simulink model "zerodiv01"  (Simulink 7.8)
settings: Solver=FixedStepDiscrete  StartTime=0.0  StopTime=10.0  FixedStep=Auto  RelTol=1e-3
settings Model: Creator=itoy  LastModifiedBy=itoy
settings DataIOCC: LimitDataPoints=off  SaveFormat=StructureWithTime  SaveOutput=off  SaveTime=off
settings OptimizationCC: OptimizeModelRefInitCode=on  LifeSpan=1
settings DebuggingCC: StrictBusMsg=Warning
settings RTWCC: SystemTargetFile=ert.tlc  GenCodeOnly=on  TemplateMakefile=ert_default_tmf  Description=Real-Time Workshop Embedded Coder  GenerateReport=on  ProcessScript=ert_make_rtw_hook  IncludeHyperlinkInReport=on  LaunchReport=on  GenerateTraceInfo=on  GenerateTraceReport=on  GenerateTraceReportSl=on  GenerateTraceReportSf=on  GenerateTraceReportEml=on
settings CodeAppCC: IgnoreCustomStorageClasses=off
settings ERTTargetCC: MultiwordLength=2048  GenerateSampleERTMain=on  ERTCustomFileTemplate=example_file_process.tlc  ConvertIfToSwitch=off  SuppressUnreachableDefaultCases=off

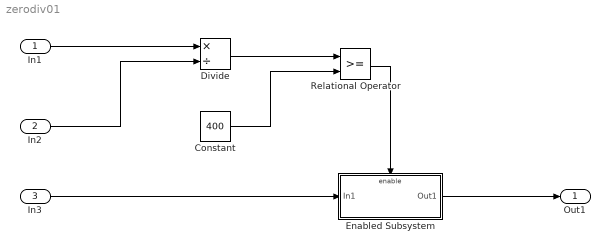
== system zerodiv01 ==
  In1 : Inport  OutMin=2  OutMax=10  OutDataTypeStr=int8
      settings: AttributesFormatString=[%<OutMax> %<OutMin>]
  In2 : Inport  Port=2  OutMin=-5  OutMax=5  OutDataTypeStr=int8
      settings: AttributesFormatString=[%<OutMax> %<OutMin>]
  In3 : Inport  Port=3  OutMin=-100  OutMax=100  OutDataTypeStr=int8
      settings: AttributesFormatString=[%<OutMax> %<OutMin>]
  Constant : Constant  Value=400
  Divide : Product  Inputs=*/
  Enabled Subsystem : Subsystem  TreatAsAtomicUnit=on
  Relational Operator : RelationalOperator  OutDataTypeStr=boolean
  Out1 : Outport
  wires:
  In1/1 -> Divide/1
  In2/1 -> Divide/2
  Divide/1 -> Relational Operator/1
  Constant/1 -> Relational Operator/2
  Relational Operator/1 -> Enabled Subsystem/Enable
  In3/1 -> Enabled Subsystem/1(In1)
  Enabled Subsystem/1(Out1) -> Out1/1

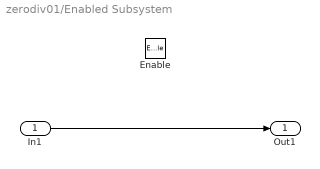
== system zerodiv01/Enabled Subsystem ==
  In1 : Inport
  Enable : EnablePort
  Out1 : Outport
  wires:
  In1/1 -> Out1/1
